simulink model "termin7simulink"  (R2022b)
settings: Solver=VariableStepAuto  StartTime=0.0  StopTime=t_simulation  MaxStep=0.1  RelTol=1e-3
values from neighbouring files (symbols this model uses):
  Cvp = cp * rop * Vp    (= 90000)    [zajeciatermin7matalb.m]
  Cvw = cp * rop * Vw    (= 150000)    [zajeciatermin7matalb.m]
  dTzad = 5    [zajeciatermin7matalb.m]
  dTzew = 0    [zajeciatermin7matalb.m]
  K = 0.003    [zajeciatermin7matalb.m]
  Kcp = (qgN*a*(TwewN-TpN))/((TwewN * (1 + a) - TzewN - a*TpN)  * (TpN - TzewN))    (= 19.6078431373)    [zajeciatermin7matalb.m]
  Kcw = qgN/(TwewN * (1 + a) - TzewN - a * TpN)    (= 235.294117647)    [zajeciatermin7matalb.m]
  Kcwp = a*Kcw    (= 58.8235294118)    [zajeciatermin7matalb.m]
  Ki = 1/Ti    (= 0.000556111667223)    [zajeciatermin7matalb.m]
  Kp = (0.9*TTp)/(K0Tp*T0Tp)    (= 763.333333333)    [zajeciatermin7matalb.m]
  qg0 = Twew0*(Kcw+Kcwp)-Tp0*Kcwp-Kcw*((Tp0*(Kcp+Kcwp)-Twew0*Kcwp)/Kcp)    (= 10000)    [zajeciatermin7matalb.m]
  t0 = 5000    [zajeciatermin7matalb.m]
  T0TpDP = 690    [zajeciatermin7matalb.m]
  Ti = 3.33*T0Tp    (= 1798.2)    [zajeciatermin7matalb.m]
  Tp0 = ((Kcw + Kcwp)*Kcp*Tzew0 + Kcwp*(qg0 + Kcw*Tzew0))/(Kcw*(Kcwp + Kcp) + Kcwp*Kcp)    (= 10)    [zajeciatermin7matalb.m]
  Twew0 = (qg0*(Kcwp + Kcp) + Tzew0*(Kcw*Kcwp + Kcw * Kcp + Kcwp * Kcp))/(Kcw*(Kcwp + Kcp) + Kcwp * Kcp)    (= 20)    [zajeciatermin7matalb.m]
  Tzad = TpN    (= 10)    [zajeciatermin7matalb.m]
  Tzew0 = TzewN    (= -20)    [zajeciatermin7matalb.m]
settings Model: Creator=huber  LastModifiedBy=huber
settings DataIOCC: ReturnWorkspaceOutputs=off

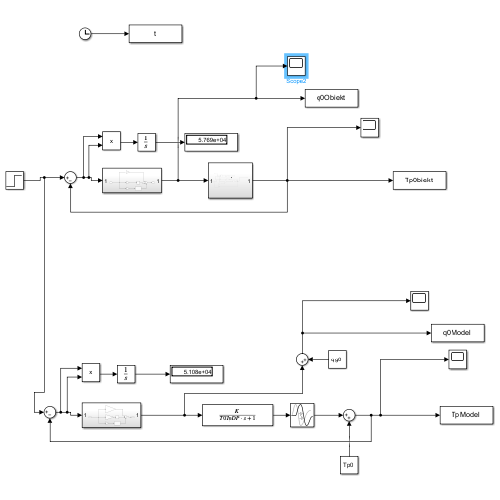
[thumbnail: Simulink's stored preview of the top-level diagram]
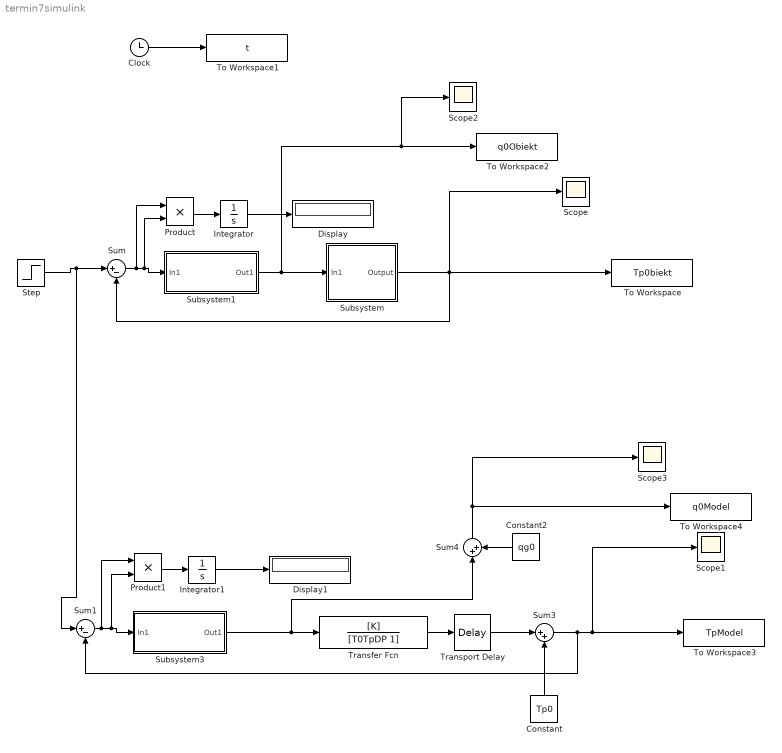
== system termin7simulink ==
  Clock : Clock
  Constant : Constant  Value=Tp0
  Constant2 : Constant  Value=qg0
  Display : Display
  Display1 : Display
  Integrator : Integrator
  Integrator1 : Integrator
  Product : Product
  Product1 : Product
  Scope{,1..3} (4 alike) : Scope
  Step : Step  Time=t0  Before=Tzad  After=Tzad + dTzad  SampleTime=0
  Subsystem : Subsystem
  Subsystem1 : Subsystem
  Subsystem3 : Subsystem
  Sum : Sum  Inputs=|+-
  Sum1 : Sum  Inputs=|+-
  Sum3 : Sum  Inputs=|++
  Sum4 : Sum  Inputs=|++
  To Workspace : ToWorkspace  VariableName=Tp0biekt  SampleTime=-1
  To Workspace1 : ToWorkspace  VariableName=t  SampleTime=-1
  To Workspace2 : ToWorkspace  VariableName=q0Obiekt  SampleTime=-1
  To Workspace3 : ToWorkspace  VariableName=TpModel  SampleTime=-1
  To Workspace4 : ToWorkspace  VariableName=q0Model  SampleTime=-1
  Transfer Fcn : TransferFcn  Numerator=[K]  Denominator=[T0TpDP 1]
  Transport Delay : TransportDelay  DelayTime=144
  wires:
  Constant/1 -> Sum3/2
  Constant2/1 -> Sum4/2
  Integrator1/1 -> Display1/1
  Subsystem3/1(Out1) -> Sum4/1, Transfer Fcn/1
  Subsystem/1(Output) -> To Workspace/1, Scope/1, Sum/2
  Step/1 -> Sum1/1, Sum/1
  Sum1/1 -> Product1/1, Product1/2, Subsystem3/1(In1)
  Subsystem1/1(Out1) -> Scope2/1, To Workspace2/1, Subsystem/1(In1)
  Integrator/1 -> Display/1
  Product1/1 -> Integrator1/1
  Clock/1 -> To Workspace1/1
  Sum/1 -> Product/1, Product/2, Subsystem1/1(In1)
  Sum4/1 -> To Workspace4/1, Scope3/1
  Transfer Fcn/1 -> Transport Delay/1
  Sum3/1 -> Sum1/2, Scope1/1, To Workspace3/1
  Transport Delay/1 -> Sum3/1
  Product/1 -> Integrator/1

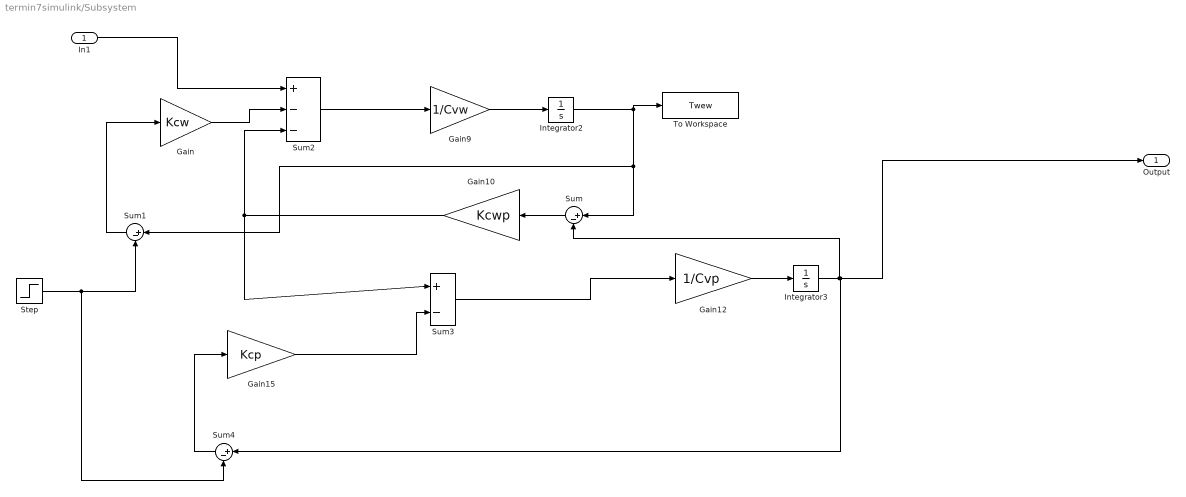
== system termin7simulink/Subsystem ==
  In1 : Inport
  Gain : Gain  Gain=Kcw
  Gain10 : Gain  Gain=Kcwp
  Gain12 : Gain  Gain=1/Cvp
  Gain15 : Gain  Gain=Kcp
  Gain9 : Gain  Gain=1/Cvw
  Integrator2 : Integrator  InitialCondition=Twew0
  Integrator3 : Integrator  InitialCondition=Tp0
  Step : Step  Time=t0  Before=Tzew0  After=Tzew0 + dTzew  SampleTime=0
  Sum{,1,3..4} (4 alike) : Sum  Inputs=|+-
  Sum2 : Sum  Inputs=+--
  To Workspace : ToWorkspace  VariableName=Twew  SampleTime=-1
  Output : Outport
  wires:
  Gain12/1 -> Integrator3/1
  Integrator2/1 -> To Workspace/1, Sum1/1, Sum/1
  Sum2/1 -> Gain9/1
  Gain9/1 -> Integrator2/1
  Gain10/1 -> Sum2/3, Sum3/1
  Integrator3/1 -> Output/1, Sum4/1, Sum/2
  Sum3/1 -> Gain12/1
  Gain15/1 -> Sum3/2
  In1/1 -> Sum2/1
  Step/1 -> Sum4/2, Sum1/2
  Gain/1 -> Sum2/2
  Sum1/1 -> Gain/1
  Sum/1 -> Gain10/1
  Sum4/1 -> Gain15/1

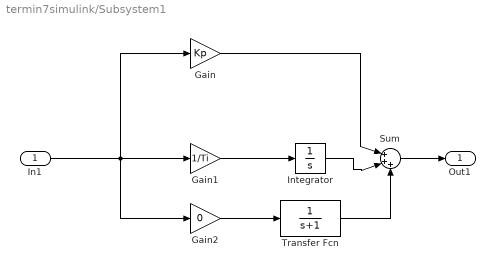
== system termin7simulink/Subsystem1 ==
  In1 : Inport
  Gain : Gain  Gain=Kp
  Gain1 : Gain  Gain=1/Ti
  Gain2 : Gain  Gain=0
  Integrator : Integrator  InitialCondition=qg0
  Sum : Sum  Inputs=|+++
  Transfer Fcn : TransferFcn  Denominator=[1 1]
  Out1 : Outport
  wires:
  In1/1 -> Gain2/1, Gain1/1, Gain/1
  Gain2/1 -> Transfer Fcn/1
  Gain/1 -> Sum/1
  Transfer Fcn/1 -> Sum/3
  Sum/1 -> Out1/1
  Gain1/1 -> Integrator/1
  Integrator/1 -> Sum/2

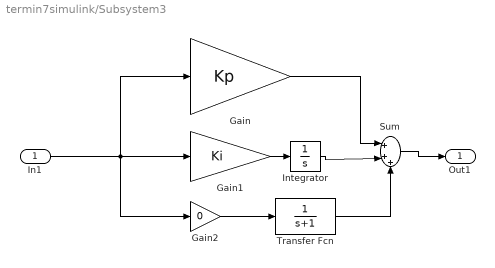
== system termin7simulink/Subsystem3 ==
  In1 : Inport
  Gain : Gain  Gain=Kp
  Gain1 : Gain  Gain=Ki
  Gain2 : Gain  Gain=0
  Integrator : Integrator
  Sum : Sum  Inputs=|+++
  Transfer Fcn : TransferFcn  Denominator=[1 1]
  Out1 : Outport
  wires:
  In1/1 -> Gain/1, Gain1/1, Gain2/1
  Gain/1 -> Sum/1
  Transfer Fcn/1 -> Sum/3
  Sum/1 -> Out1/1
  Gain2/1 -> Transfer Fcn/1
  Gain1/1 -> Integrator/1
  Integrator/1 -> Sum/2
